simulink subsystem "In_Plane_Model"  (R2025b)
settings: Solver=VariableStepAuto  StartTime=0.0  StopTime=10.0  RelTol=1e-3
undefined symbols (not defined in the file): AeroLiftCff, AeroLongDrgCff, AeroMotoEffctArea, AeroPitchMomentCff, AeroPitchMomentLngth, AeroRltWindAngVect, AeroSideFrcCff, AeroYawMomentCff, aMode, BrkFrntBrkActrBore, BrkFrntBrkActrPrsBpt, BrkFrntBrkPadMeanRadius, BrkFrntBrkTrqTbl, BrkFrntIntrnRadius, BrkFrntKinFricCff, BrkFrntPadNum, BrkFrntShoePinToDrumCntrDst, BrkFrntShoePinToFrcAppDst, BrkFrntShoePinToPadEndAng, BrkFrntShoePinToPadStartAng, BrkFrntStcFricCff, BrkFrntWhlSpdBpt, BrkRearBrkActrBore, BrkRearBrkActrPrsBpt, BrkRearBrkPadMeanRadius, BrkRearBrkTrqTbl, BrkRearIntrnRadius, BrkRearKinFricCff, BrkRearPadNum, BrkRearShoePinToDrumCntrDst, BrkRearShoePinToFrcAppDst, BrkRearShoePinToPadEndAng, BrkRearShoePinToPadStartAng, BrkRearStcFricCff, BrkRearWhlSpdBpt, EnvAbsPrs, EnvAirTemp, FrkFrL0, FrmAng0, g, GasCnst, InitFrkLngth, InitMainFrmPitchAng, InitRearArmPitchAng, InitRearCntctPtchLatVel, InitRearCntctPtchLongVel, InitRearCntctPtchY, InitRearCntctPtchZ, InitRollAng, InitYawAng, MotoFrmLngth, MotoFrmMass, MotoGrvty, MotoLatOfst, MotoLongOfst, MotoLowrFrntFrkMass, MotoPtchOfst, MotoRearArmLngth, MotoRearArmMass, MotoRollOfst ... (+25)
libraries: sm_lib x309, nesl_utility_internal x158, nesl_utility x7, autolibsharedcoupling x6, vehdynlibtire x6, sharedtransform x4, shared6dof x1, matrix_library x1, vehdynlibeomcommon x1
(part 1 of 10)
settings Model: Creator=The MathWorks, Inc.  LastModifiedBy=Omen
settings RTWCC: GPUComputeCapability=3.5

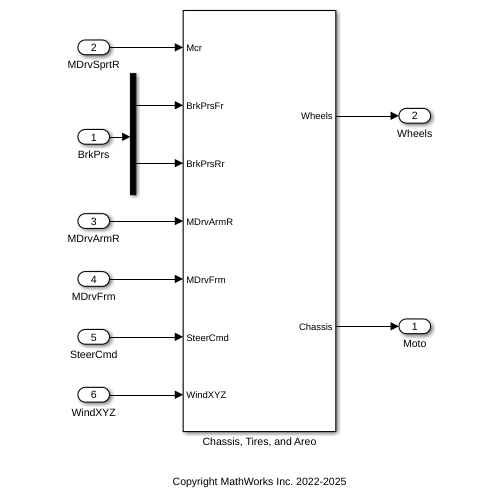
[thumbnail: Simulink's stored preview of the top-level diagram]
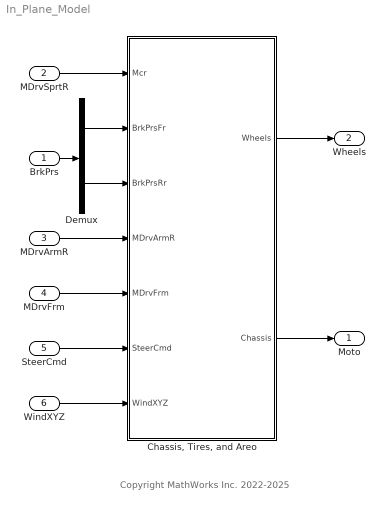
== system In_Plane_Model ==
  note: Copyright MathWorks Inc. 2022-2025
  BrkPrs : Inport
  MDrvSprtR : Inport  Port=2
  MDrvArmR : Inport  Port=3
  MDrvFrm : Inport  Port=4
  SteerCmd : Inport  Port=5
  WindXYZ : Inport  Port=6
  "Chassis, Tires, and Areo" : Subsystem
  Demux : Demux  Outputs=2
  Moto : Outport
  Wheels : Outport  Port=2
  wires:
  BrkPrs/1 -> Demux/1
  "Chassis, Tires, and Areo"/1(Wheels) -> Wheels/1
  Demux/2 -> "Chassis, Tires, and Areo"/3(BrkPrsRr)
  Demux/1 -> "Chassis, Tires, and Areo"/2(BrkPrsFr)
  "Chassis, Tires, and Areo"/2(Chassis) -> Moto/1
  MDrvSprtR/1 -> "Chassis, Tires, and Areo"/1(Mcr)
  MDrvFrm/1 -> "Chassis, Tires, and Areo"/5(MDrvFrm)
  MDrvArmR/1 -> "Chassis, Tires, and Areo"/4(MDrvArmR)
  SteerCmd/1 -> "Chassis, Tires, and Areo"/6(SteerCmd)
  WindXYZ/1 -> "Chassis, Tires, and Areo"/7(WindXYZ)

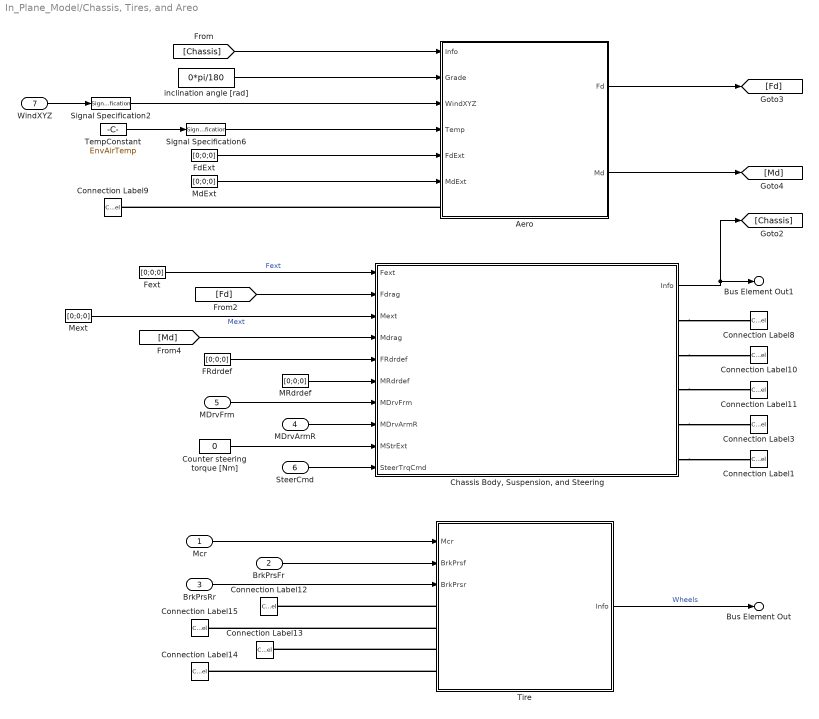
== system In_Plane_Model/Chassis, Tires, and Areo ==
  Mcr : Inport
  BrkPrsFr : Inport  Port=2
  BrkPrsRr : Inport  Port=3
  MDrvArmR : Inport  Port=4
  MDrvFrm : Inport  Port=5
  SteerCmd : Inport  Port=6
  WindXYZ : Inport  Port=7
  Aero : Subsystem  Variant=on  VariantControlMode=label  VariantControl=Choice  LabelModeActiveChoice=None
  "Chassis Body, Suspension, and Steering" : Subsystem
  Connection Label1 : ConnectionLabel  Label=WhlHubFr_B
  Connection Label10 : ConnectionLabel  Label=WhlHubRr_F
  Connection Label11 : ConnectionLabel  Label=WhlHubFr_F
  Connection Label12 : ConnectionLabel  Label=WhlHubFr_B
  Connection Label13 : ConnectionLabel  Label=WhlHubRr_B
  Connection Label14 : ConnectionLabel  Label=WhlHubRr_F
  Connection Label15 : ConnectionLabel  Label=WhlHubFr_F
  Connection Label3 : ConnectionLabel  Label=WhlHubRr_B
  Connection Label8 : ConnectionLabel  Label=AeroFrame_Frm
  Connection Label9 : ConnectionLabel  Label=AeroFrame_Frm
  Counter steering torque [Nm] : Constant  Value=0
  FRdrdef : Constant  Value=[0;0;0]
  FdExt : Constant  Value=[0;0;0]
  Fext : Constant  Value=[0;0;0]
  MRdrdef : Constant  Value=[0;0;0]
  MdExt : Constant  Value=[0;0;0]
  Mext : Constant  Value=[0;0;0]
  Signal Specification2 : SignalSpecification  Unit=m/s
  Signal Specification6 : SignalSpecification  Unit=K
  TempConstant : Constant  Value=EnvAirTemp
  Tire : Subsystem
  inclination angle [rad] : Constant  Value=0*pi/180
  Bus Element Out : Outport  PortName=Wheels
  Bus Element Out1 : Outport  Port=2  PortName=Chassis
  wires:
  SteerCmd/1 -> "Chassis Body, Suspension, and Steering"/10(SteerTrqCmd)
  Counter steering torque [Nm]/1 -> "Chassis Body, Suspension, and Steering"/9(MStrExt)
  MDrvArmR/1 -> "Chassis Body, Suspension, and Steering"/8(MDrvArmR)
  MDrvFrm/1 -> "Chassis Body, Suspension, and Steering"/7(MDrvFrm)
  [Chassis] -> Aero/1(Info)
  "Chassis Body, Suspension, and Steering"/1(Info) -> [Chassis], Bus Element Out1/1
  Tire/1(Info) -> Bus Element Out/1  "Wheels"
  BrkPrsRr/1 -> Tire/3(BrkPrsr)
  Mcr/1 -> Tire/1(Mcr)
  BrkPrsFr/1 -> Tire/2(BrkPrsf)
  MRdrdef/1 -> "Chassis Body, Suspension, and Steering"/6(MRdrdef)
  FRdrdef/1 -> "Chassis Body, Suspension, and Steering"/5(FRdrdef)
  [Md] -> "Chassis Body, Suspension, and Steering"/4(Mdrag)
  [Fd] -> "Chassis Body, Suspension, and Steering"/2(Fdrag)
  Fext/1 -> "Chassis Body, Suspension, and Steering"/1(Fext)  "Fext"
  Mext/1 -> "Chassis Body, Suspension, and Steering"/3(Mext)  "Mext"
  Aero/2(Md) -> [Md]
  Aero/1(Fd) -> [Fd]
  Signal Specification6/1 -> Aero/4(Temp)
  Signal Specification2/1 -> Aero/3(WindXYZ)
  FdExt/1 -> Aero/5(FdExt)
  WindXYZ/1 -> Signal Specification2/1
  inclination angle [rad]/1 -> Aero/2(Grade)
  TempConstant/1 -> Signal Specification6/1
  MdExt/1 -> Aero/6(MdExt)
  connections:
  Tire/LConn3 -- Connection Label13/LConn1
  "Chassis Body, Suspension, and Steering"/RConn4 -- Connection Label3/LConn1
  "Chassis Body, Suspension, and Steering"/RConn2 -- Connection Label10/LConn1
  "Chassis Body, Suspension, and Steering"/RConn3 -- Connection Label11/LConn1
  "Chassis Body, Suspension, and Steering"/RConn1 -- Connection Label8/LConn1
  "Chassis Body, Suspension, and Steering"/RConn5 -- Connection Label1/LConn1
  Tire/LConn4 -- Connection Label14/LConn1
  Tire/LConn1 -- Connection Label12/LConn1
  Tire/LConn2 -- Connection Label15/LConn1
  Aero/LConn1 -- Connection Label9/LConn1

== system In_Plane_Model/Chassis, Tires, and Areo/Aero ==
  Info : Inport
  Grade : Inport  Port=2
  WindXYZ : Inport  Port=3
  Temp : Inport  Port=4
  FdExt : Inport  Port=5
  MdExt : Inport  Port=6
  External : Subsystem  VariantControl=External
  None : Subsystem  VariantControl=None
  Standard Ambient : Subsystem  VariantControl=Standard Ambient
  AeroFrame_Frm : PMIOPort  Side=Left
  Fd : Outport
  Md : Outport  Port=2

== system In_Plane_Model/Chassis, Tires, and Areo/Chassis Body, Suspension, and Steering ==
  Fext : Inport
  Fdrag : Inport  Port=2
  Mext : Inport  Port=3
  Mdrag : Inport  Port=4
  FRdrdef : Inport  Port=5
  MRdrdef : Inport  Port=6
  MDrvFrm : Inport  Port=7
  MDrvArmR : Inport  Port=8
  MStrExt : Inport  Port=9
  SteerTrqCmd : Inport  Port=10
  CHASSIS : Subsystem
  FSusfin : Ground
  MStrDmpin : Ground
  MSusrin : Ground
  Signal routine : Subsystem
  WhlHubFr_F : PMIOPort  Side=Right
  WhlHubRr_F : PMIOPort  Port=2  Side=Right
  AeroFrame_Frm : PMIOPort  Port=3  Side=Right
  WhlHubRr_B : PMIOPort  Port=4  Side=Right
  WhlHubFr_B : PMIOPort  Port=5  Side=Right
  Info : Outport
  wires:
  Mdrag/1 -> [Md], CHASSIS/6(Mdrag)
  Fdrag/1 -> [Fd], CHASSIS/5(Fdrag)  "Fdrag"
  MStrExt/1 -> CHASSIS/8(MStrExt)
  CHASSIS/16(GeomInfo) -> Signal routine/19(GeomInfo)
  MStrDmpin/1 -> CHASSIS/13(MStrDmpin)
  MRdrdef/1 -> CHASSIS/12(MRdrdef)
  FRdrdef/1 -> CHASSIS/11(FRdrdef)
  CHASSIS/15(Q,A,V,P_Rdr) -> Signal routine/18(Q,A,V,P_Rdr)
  FSusfin/1 -> CHASSIS/10(FSusfin)
  MSusrin/1 -> CHASSIS/9(MSusrin)
  CHASSIS/14(Grvty) -> Signal routine/17(Grvty)
  CHASSIS/13(Fext_BF) -> Signal routine/16(Fext_BF)
  CHASSIS/4(WhlFrCpY) -> Signal routine/7(WhlFrCpY)
  Mext/1 -> CHASSIS/2(Mext), [Mext]  "Mext"
  CHASSIS/12(A,V,P_str) -> Signal routine/15(SteerAng)
  CHASSIS/3(WhlRrCpY) -> Signal routine/6(WhlRrCpY)
  SteerTrqCmd/1 -> CHASSIS/7(MSteer)
  [Fd] -> Signal routine/2(Fd)
  [Md] -> Signal routine/3(Md)
  MDrvArmR/1 -> CHASSIS/3(MDrvArmR)  "MDrvArmR"
  MDrvFrm/1 -> CHASSIS/4(MDrvFrm)  "MDrvFrm"
  Signal routine/1(Info) -> Info/1  "ChassisInfo"
  CHASSIS/11(FrkFz) -> Signal routine/14(Frk)
  CHASSIS/10(ShkMy) -> Signal routine/13(Shk)
  CHASSIS/9(Lfrk) -> Signal routine/12(Lfrk)
  CHASSIS/8(A,V,P_FrmAng) -> Signal routine/11(FrmAng)
  CHASSIS/7(ArmRrAng) -> Signal routine/10(ArmRrAng)
  CHASSIS/6(WhlFrCpZ) -> Signal routine/9(WhlFrCpZ)
  CHASSIS/5(WhlRrCpZ) -> Signal routine/8(WhlRrCpZ)
  CHASSIS/2(WhlFrCpX) -> Signal routine/5(WhlFrCpX)
  CHASSIS/1(WhlRrCpX) -> Signal routine/4(WhlRrCpX)
  [Mext] -> Signal routine/1(Mext)
  Fext/1 -> CHASSIS/1(Fext)  "Fext"
  connections:
  CHASSIS/RConn9 -- AeroFrame_Frm/RConn1
  Signal routine/LConn1 -- CHASSIS/RConn1
  Signal routine/LConn2 -- CHASSIS/RConn2
  Signal routine/LConn7 -- CHASSIS/RConn7
  CHASSIS/RConn6 -- Signal routine/LConn6
  CHASSIS/RConn5 -- Signal routine/LConn5
  CHASSIS/RConn3 -- Signal routine/LConn3
  WhlHubRr_F/RConn1 -- CHASSIS/RConn11
  WhlHubFr_F/RConn1 -- CHASSIS/RConn10
  Signal routine/LConn8 -- CHASSIS/RConn8
  WhlHubRr_B/RConn1 -- CHASSIS/LConn1
  Signal routine/LConn4 -- CHASSIS/RConn4
  CHASSIS/LConn2 -- WhlHubFr_B/RConn1

== system In_Plane_Model/Chassis, Tires, and Areo/Tire ==
  Mcr : Inport
  BrkPrsf : Inport  Port=2
  BrkPrsr : Inport  Port=3
  Bus Creator : BusCreator  Inputs=2
  Front Tire : Subsystem  Variant=on  VariantControlMode=label  LabelModeActiveChoice=Linear Front SSC Tire
  MWhf : Ground
  MWhr : Ground
  Mcrf : Ground
  Rear Tire : Subsystem  Variant=on  VariantControlMode=label  LabelModeActiveChoice=Linear Rear SSC Tire
  Terminator{,1..11} (12 alike) : Terminator
  HubJointFr_B : PMIOPort  Side=Left
  HubJointFr_F : PMIOPort  Port=2  Side=Left
  HubJointRr_B : PMIOPort  Port=3  Side=Left
  HubJointRr_F : PMIOPort  Port=4  Side=Left
  Info : Outport
  wires:
  Bus Creator/1 -> Info/1
  Front Tire/4(Fz) -> Terminator2/1  "Fz"
  Mcrf/1 -> Front Tire/2(Mcr)
  Front Tire/2(Fx) -> Terminator/1  "Fx"
  Front Tire/6(My) -> Terminator4/1  "My"
  Front Tire/7(Mz) -> Terminator5/1  "Mz"
  Front Tire/5(Mx) -> Terminator3/1  "Mx"
  Front Tire/1(Info) -> Bus Creator/1  "FrontTire"
  BrkPrsf/1 -> Front Tire/3(BrkPrs)
  Front Tire/3(Fy) -> Terminator1/1  "Fy"
  Rear Tire/3(Fy) -> Terminator7/1  "Fy"
  Rear Tire/2(Fx) -> Terminator6/1  "Fx"
  Rear Tire/4(Fz) -> Terminator8/1  "Fz"
  Rear Tire/7(Mz) -> Terminator11/1  "Mz"
  Rear Tire/5(Mx) -> Terminator9/1  "Mx"
  Rear Tire/6(My) -> Terminator10/1  "My"
  Rear Tire/1(Info) -> Bus Creator/2  "RearTire"
  MWhf/1 -> Front Tire/1(MWh)
  BrkPrsr/1 -> Rear Tire/3(BrkPrs)
  MWhr/1 -> Rear Tire/1(MWh)
  Mcr/1 -> Rear Tire/2(Mcr)
  connections:
  Front Tire/LConn1 -- HubJointFr_B/RConn1
  Front Tire/LConn2 -- HubJointFr_F/RConn1
  Rear Tire/LConn2 -- HubJointRr_F/RConn1
  Rear Tire/LConn1 -- HubJointRr_B/RConn1

== system In_Plane_Model/Chassis, Tires, and Areo/Aero/External ==
  FdExt : Inport
  MdExt : Inport  Port=2
  Fd : Outport
  Md : Outport  Port=2
  wires:
  MdExt/1 -> Md/1
  FdExt/1 -> Fd/1

== system In_Plane_Model/Chassis, Tires, and Areo/Aero/None ==
  Constant : Constant  Value=[0 0 0]
  Constant1 : Constant  Value=[0 0 0]
  Fd : Outport
  Md : Outport  Port=2
  wires:
  Constant/1 -> Fd/1
  Constant1/1 -> Md/1

== system In_Plane_Model/Chassis, Tires, and Areo/Aero/Standard Ambient ==
  Info : Inport
  Grade : Inport  Port=2  Unit=rad
  WindXYZ : Inport  Port=3  PortDimensions=3
  Temp : Inport  Port=4
  Bus Selector6 : BusSelector  OutputSignals=Frame.InertFrm.Cg.Ang.theta
  Drag Force : Subsystem  mask{A=AeroMotoEffctArea, beta_w=AeroRltWindAngVect, Cd=AeroLongDrgCff, Cs=AeroSideFrcCff, Cl=AeroLiftCff, Cpm=AeroPitchMomentCff, Lcpm=AeroPitchMomentLngth, Crm=[0,0], Cym=AeroYawMomentCff, R=GasCnst, Pabs=EnvAbsPrs}
      mask prompts: A "Effective area, A [m^s2]:"; beta_w "Relative wind angle vector, beta_w [rad]:"; Cd "Longitudinal drag coefficient, Cd [-]:"; Cs "Side force coefficient data, Cs [-]:"; Cl "Lift coefficient, Cl [-]:"; Cpm "Pitch moment coefficient, Cpm [-]:"; Lcpm "Pitch moment length, Lcpm"; Crm "Roll moment coefficient data, Crm [-]:"; Cym "Yaw moment coefficient data, Cym [-]:"; R "Gas constant, R [J/(kg*K)]:"; Pabs "Absoulte pressure, Pabs [Pa]:"
  Mux6 : Mux  Inputs=3
  Sensor_Frm : Subsystem
  Subtract : Sum  Inputs=--
  Unary Minus : UnaryMinus
  Unary Minus1 : UnaryMinus
  rotation : Subsystem  TreatAsAtomicUnit=on  mask(Rotation){aMode=aMode}
  AeroFrame_Frm : PMIOPort  Side=Left
  Fd : Outport
  Md : Outport  Port=2
  wires:
  Sensor_Frm/3(Vz_vf) -> Mux6/3
  Temp/1 -> Drag Force/3(T)
  Sensor_Frm/1(Vx_vf) -> Mux6/1
  Mux6/1 -> Drag Force/1(Body Axis Vel)
  WindXYZ/1 -> rotation/1(X)
  Bus Selector6/1 -> Subtract/1  "<theta>"
  Sensor_Frm/2(Vy_vf) -> Mux6/2
  Info/1 -> Bus Selector6/1
  Drag Force/1(Fd) -> Unary Minus1/1
  Drag Force/2(Md) -> Unary Minus/1
  Subtract/1 -> rotation/2(theta)
  Grade/1 -> Subtract/2
  rotation/1(x) -> Drag Force/2(Body Axis Wind)
  Unary Minus1/1 -> Fd/1
  Unary Minus/1 -> Md/1
  connections:
  AeroFrame_Frm/RConn1 -- Sensor_Frm/LConn1

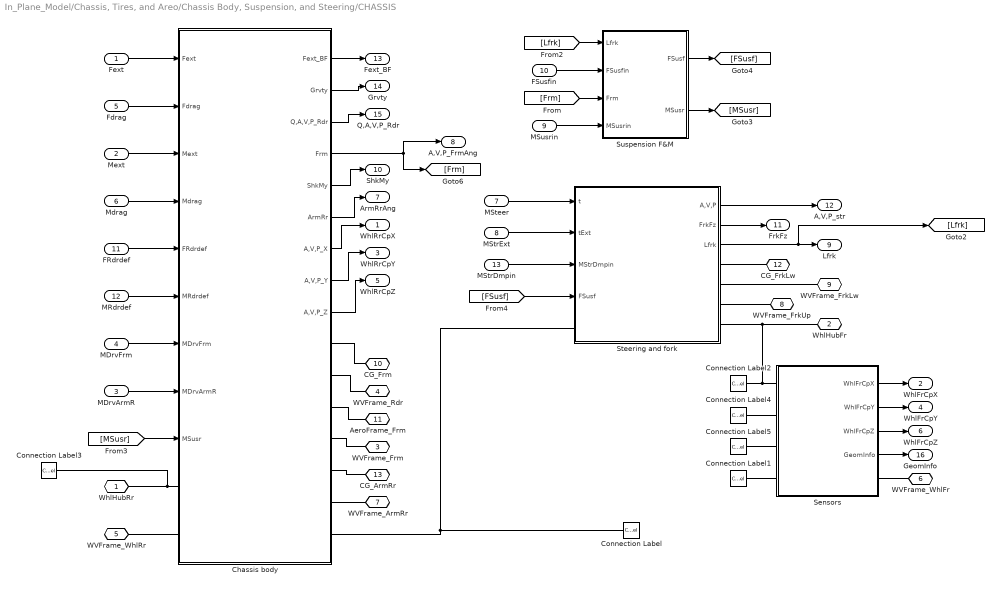
== system In_Plane_Model/Chassis, Tires, and Areo/Chassis Body, Suspension, and Steering/CHASSIS ==
  Fext : Inport
  Mext : Inport  Port=2
  MDrvArmR : Inport  Port=3
  MDrvFrm : Inport  Port=4
  Fdrag : Inport  Port=5
  Mdrag : Inport  Port=6
  MSteer : Inport  Port=7
  MStrExt : Inport  Port=8
  MSusrin : Inport  Port=9
  FSusfin : Inport  Port=10
  FRdrdef : Inport  Port=11
  MRdrdef : Inport  Port=12
  MStrDmpin : Inport  Port=13
  Chassis body : Subsystem
  Connection Label : ConnectionLabel  Label=pivo
  Connection Label1 : ConnectionLabel  Label=pivo
  Connection Label2 : ConnectionLabel  Label=HubFr
  Connection Label3 : ConnectionLabel  Label=HubRr
  Connection Label4 : ConnectionLabel  Label=HubRr
  Connection Label5 : ConnectionLabel  Label=HubFr
  Sensors : Subsystem
  Steering and fork : Subsystem
  Suspension F&M : Subsystem
  WhlHubRr : PMIOPort  Side=Left
  WhlHubFr : PMIOPort  Port=2  Side=Left
  WVFrame_Frm : PMIOPort  Port=3  Side=Right
  WVFrame_Rdr : PMIOPort  Port=4  Side=Right
  WVFrame_WhlRr : PMIOPort  Port=5  Side=Right
  WVFrame_WhlFr : PMIOPort  Port=6  Side=Right
  WVFrame_ArmRr : PMIOPort  Port=7  Side=Right
  WVFrame_FrkUp : PMIOPort  Port=8  Side=Right
  WVFrame_FrkLw : PMIOPort  Port=9  Side=Right
  CG_Frm : PMIOPort  Port=10  Side=Right
  AeroFrame_Frm : PMIOPort  Port=11  Side=Right
  CG_FrkLw : PMIOPort  Port=12  Side=Right
  CG_ArmRr : PMIOPort  Port=13  Side=Right
  WhlRrCpX : Outport
  WhlFrCpX : Outport  Port=2
  WhlRrCpY : Outport  Port=3
  WhlFrCpY : Outport  Port=4
  WhlRrCpZ : Outport  Port=5
  WhlFrCpZ : Outport  Port=6
  ArmRrAng : Outport  Port=7
  A,V,P_FrmAng : Outport  Port=8
  Lfrk : Outport  Port=9
  ShkMy : Outport  Port=10
  FrkFz : Outport  Port=11
  A,V,P_str : Outport  Port=12
  Fext_BF : Outport  Port=13
  Grvty : Outport  Port=14
  Q,A,V,P_Rdr : Outport  Port=15
  GeomInfo : Outport  Port=16
  wires:
  Chassis body/9(A,V,P_Z) -> WhlRrCpZ/1
  Chassis body/8(A,V,P_Y) -> WhlRrCpY/1
  Chassis body/7(A,V,P_X) -> WhlRrCpX/1
  Chassis body/6(ArmRr) -> ArmRrAng/1
  Chassis body/5(ShkMy) -> ShkMy/1
  Chassis body/3(Q,A,V,P_Rdr) -> Q,A,V,P_Rdr/1
  Chassis body/2(Grvty) -> Grvty/1
  Chassis body/1(Fext_BF) -> Fext_BF/1
  [MSusr] -> Chassis body/9(MSusr)
  MDrvArmR/1 -> Chassis body/8(MDrvArmR)
  MDrvFrm/1 -> Chassis body/7(MDrvFrm)
  MRdrdef/1 -> Chassis body/6(MRdrdef)
  FRdrdef/1 -> Chassis body/5(FRdrdef)
  Mdrag/1 -> Chassis body/4(Mdrag)
  Mext/1 -> Chassis body/3(Mext)
  Fdrag/1 -> Chassis body/2(Fdrag)
  Fext/1 -> Chassis body/1(Fext)
  Chassis body/4(Frm) -> A,V,P_FrmAng/1, [Frm]
  Steering and fork/2(FrkFz) -> FrkFz/1
  Steering and fork/1(A,V,P) -> A,V,P_str/1
  [FSusf] -> Steering and fork/4(FSusf)
  MStrDmpin/1 -> Steering and fork/3(MStrDmpin)
  MStrExt/1 -> Steering and fork/2(tExt)
  MSteer/1 -> Steering and fork/1(t)
  Steering and fork/3(Lfrk) -> Lfrk/1, [Lfrk]
  Sensors/4(GeomInfo) -> GeomInfo/1
  Sensors/3(WhlFrCpZ) -> WhlFrCpZ/1
  Sensors/2(WhlFrCpY) -> WhlFrCpY/1
  Sensors/1(WhlFrCpX) -> WhlFrCpX/1
  Suspension F&M/2(MSusr) -> [MSusr]
  Suspension F&M/1(FSusf) -> [FSusf]
  MSusrin/1 -> Suspension F&M/4(MSusrin)
  [Frm] -> Suspension F&M/3(Frm)
  FSusfin/1 -> Suspension F&M/2(FSusfin)
  [Lfrk] -> Suspension F&M/1(Lfrk)
  connections:
  WVFrame_WhlRr/RConn1 -- Chassis body/LConn2
  Chassis body/RConn6 -- WVFrame_ArmRr/RConn1
  Chassis body/RConn5 -- CG_ArmRr/RConn1
  WVFrame_Frm/RConn1 -- Chassis body/RConn4
  AeroFrame_Frm/RConn1 -- Chassis body/RConn3
  Chassis body/RConn2 -- WVFrame_Rdr/RConn1
  CG_Frm/RConn1 -- Chassis body/RConn1
  Chassis body/LConn1 -- WhlHubRr/RConn1 -- Connection Label3/LConn1
  Chassis body/RConn7 -- Steering and fork/LConn1 -- Connection Label/LConn1
  Steering and fork/RConn3 -- WVFrame_FrkUp/RConn1
  Steering and fork/RConn2 -- WVFrame_FrkLw/RConn1
  Steering and fork/RConn1 -- CG_FrkLw/RConn1
  Sensors/LConn4 -- Connection Label1/LConn1
  Sensors/LConn3 -- Connection Label5/LConn1
  Connection Label4/LConn1 -- Sensors/LConn2
  Sensors/RConn1 -- WVFrame_WhlFr/RConn1
  WhlHubFr/RConn1 -- Steering and fork/RConn4 -- Sensors/LConn1 -- Connection Label2/LConn1

== system In_Plane_Model/Chassis, Tires, and Areo/Chassis Body, Suspension, and Steering/Signal routine ==
  Mext : Inport
  Fd : Inport  Port=2
  Md : Inport  Port=3
  WhlRrCpX : Inport  Port=4
  WhlFrCpX : Inport  Port=5
  WhlRrCpY : Inport  Port=6
  WhlFrCpY : Inport  Port=7
  WhlRrCpZ : Inport  Port=8
  WhlFrCpZ : Inport  Port=9
  ArmRrAng : Inport  Port=10
  FrmAng : Inport  Port=11
  Lfrk : Inport  Port=12
  Shk : Inport  Port=13
  Frk : Inport  Port=14
  SteerAng : Inport  Port=15
  Fext_BF : Inport  Port=16
  Grvty : Inport  Port=17
  Q,A,V,P_Rdr : Inport  Port=18
  GeomInfo : Inport  Port=19
  Ancillary_sub : Subsystem
  Bus Creator12 : BusCreator  Inputs=8
  Geom : Subsystem
  Info_sub : Subsystem
      settings: PortSchema="{\"entries\":[{\"content\":{\"sides\":[{\"content\":{\"connectorIds\":[\"LConn1\",\"In1\",\"In2\",\"In3\",\"In4\",\"In5\",\"In6\"]},\"type\":\"ConnectorPlacement.EquallySpacedRectSide\",\"uuid\":\"4ecbd4ae-1654-4997-9989-88e0c36cbdd4\"},{\"content\":{\"connectorIds\":[\"Out1\"],\"side\":\"RIGHT\"},\"type\":\"ConnectorPlacement.EquallySpacedRectSide\",\"uuid\":\"f0d457c7-b83f-4f98-93cd-bb44a09287fe\"},{\"content\":{\"side\":\"TOP\"},\"type\":\"ConnectorPlacement.EquallySpacedRectSide\",\"uuid\":\"b5011b05-5a79-4eec-86a1-ae828fee4e52\"}]},\"type\":\"ConnectorPlacement.EquallySpacedConnector\",\"uuid\":\"9f66f65c-095d-49d5-95d1-46193111b387\"}],\"packageUris\":[\"http://schema.mathworks.com/mf0/Connector/R2020b\"],\"version\":\"1.0\"}"
  Subsystem Info Busses : Subsystem
  WVFrame_Frm : PMIOPort  Side=Left
  WVFrame_Rdr : PMIOPort  Port=2  Side=Left
  WVFrame_WhlRr : PMIOPort  Port=3  Side=Left
  WVFrame_WhlFr : PMIOPort  Port=4  Side=Left
  WVFrame_ArmRr : PMIOPort  Port=5  Side=Left
  WVFrame_FrkUp : PMIOPort  Port=6  Side=Left
  WVFrame_FrkLw : PMIOPort  Port=7  Side=Left
  CG_Frm : PMIOPort  Port=8  Side=Left
  Info : Outport
  wires:
  Subsystem Info Busses/7(Rdr) -> Bus Creator12/7  "Rdr"
  Geom/1(Geom) -> Bus Creator12/8  "Geom"
  GeomInfo/1 -> Geom/1(GeomInfo)
  Q,A,V,P_Rdr/1 -> Ancillary_sub/13(Q,A,V,P_Rdr)
  Fext_BF/1 -> Info_sub/1(Fext_BF)
  FrmAng/1 -> Ancillary_sub/8(FrmAng)
  Subsystem Info Busses/6(Steer) -> Bus Creator12/6  "Steer"
  SteerAng/1 -> Ancillary_sub/12(SteerAng), Geom/2(SteerAng)
  WhlFrCpY/1 -> Ancillary_sub/4(WhlFrCpY)
  WhlRrCpY/1 -> Ancillary_sub/3(WhlRrCpY)
  Subsystem Info Busses/4(Fork) -> Bus Creator12/4  "Fork"
  Info_sub/1(Frame) -> Bus Creator12/1  "Frame"
  Subsystem Info Busses/1(Frm) -> Info_sub/6(Genrl)  "Genrl"
  Subsystem Info Busses/5(Susp) -> Bus Creator12/5  "Susp"
  Subsystem Info Busses/3(RearArm) -> Bus Creator12/3  "RearArm"
  Subsystem Info Busses/2(Whl) -> Bus Creator12/2  "Whl"
  Fd/1 -> Info_sub/3(Fd)
  Md/1 -> Info_sub/4(Md)
  Frk/1 -> Ancillary_sub/11(Frk)
  Lfrk/1 -> Ancillary_sub/9(Lfrk)
  Shk/1 -> Ancillary_sub/10(Shk)
  WhlFrCpZ/1 -> Ancillary_sub/6(WhlFrCpZ)
  ArmRrAng/1 -> Ancillary_sub/7(ArmRrAng)
  WhlRrCpZ/1 -> Ancillary_sub/5(WhlRrCpZ)
  WhlFrCpX/1 -> Ancillary_sub/2(WhlFrCpX)
  WhlRrCpX/1 -> Ancillary_sub/1(WhlRrCpX)
  Bus Creator12/1 -> Info/1  "Info"
  Grvty/1 -> Info_sub/2(Fg)
  Mext/1 -> Info_sub/5(Mext)
  Ancillary_sub/1(Ancillary) -> Subsystem Info Busses/1(Info In)  "Ancillary"
  connections:
  Ancillary_sub/LConn7 -- WVFrame_Frm/RConn1
  WVFrame_Rdr/RConn1 -- Ancillary_sub/LConn4
  Ancillary_sub/LConn6 -- WVFrame_FrkLw/RConn1
  WVFrame_WhlRr/RConn1 -- Ancillary_sub/LConn1
  Ancillary_sub/LConn2 -- WVFrame_WhlFr/RConn1
  Ancillary_sub/LConn3 -- WVFrame_ArmRr/RConn1
  Ancillary_sub/LConn5 -- WVFrame_FrkUp/RConn1
  CG_Frm/RConn1 -- Info_sub/LConn1

== system In_Plane_Model/Chassis, Tires, and Areo/Tire/Front Tire ==
  note: 1) Add Subsystem or Model blocks as valid variant choices.
      | 2) You cannot connect blocks at this level. At simulation, connectivity is automatically
      | determined, based on the active variant and port name matching.
  MWh : Inport
  Mcr : Inport  Port=2
  BrkPrs : Inport  Port=3
  Linear Front SSC Tire : Subsystem  VariantControl=Linear Front SSC Tire  mask{BrakeTypePanel=Disc, FrictionTypePanel=Linear, VDeflectionTypePanel=Simple spring and damper, kx=TireFrntBrkDrvStf, kyl=TireFrntCrnrStf, kyc=TireFrntCamberStf, mu_static=BrkFrntStcFricCff, mu_kinetic=BrkFrntKinFricCff, drum_abore=BrkFrntBrkActrBore, drum_a=BrkFrntShoePinToDrumCntrDst, drum_c=BrkFrntShoePinToFrcAppDst, drum_r=BrkFrntIntrnRadius, drum_theta1=BrkFrntShoePinToPadStartAng, drum_theta2=BrkFrntShoePinToPadEndAng, disk_abore=BrkFrntBrkActrBore, Rm=BrkFrntBrkPadMeanRadius, num_pads=BrkFrntPadNum, brake_p_bpt=BrkFrntBrkActrPrsBpt, brake_n_bpt=BrkFrntWhlSpdBpt, f_brake_t=BrkFrntBrkTrqTbl, kz=TireFrntVertStf, cz=TireFrntVertDamp, WhlMass=TireFrntWhlMass, whlInert=TireFrntWhlInert, RWhl=TireFrntWhlRadius, omegao=-InitRearCntctPtchLongVel/TireFrntWhlRadius, aMode=2}
      mask prompts: BrakeTypePanel "Brake type:"; FrictionTypePanel "Friction model type:"; VDeflectionTypePanel "Vertical Deflection model type:"; kx "Braking/Driving stiffness, kx [-]:"; kyl "Cornering stiffness, kyl [-]:"; kyc "Camber stiffness, kyc [-]:"; mu_static "Static friction coefficient, mu_static []:"; mu_kinetic "Kinetic friction coefficient, mu_kinetic []:"; drum_abore "Drum brake actuator bore, drum_abore [m]:"; drum_a "Shoe pin to drum center distance, drum_a [m]:"; drum_c "Shoe pin center to force application point distance, drum_c [m]:"; drum_r "Drum internal radius, drum_r [m]:"; drum_theta1 "Shoe pin to pad start angle, drum_theta1 [deg]:"; drum_theta2 "Shoe pin to pad end angle, drum_theta2 [deg]:"; disk_abore "Disc brake actuator bore, disk_abore [m]:"; Rm "Brake pad mean radius, Rm [m]:"; num_pads "Number of brake pads, num_pads []:"; brake_p_bpt "Brake actuator pressure breakpoints, brake_p_bpt [bar]:"; brake_n_bpt "Wheel speed breakpoints, brake_n_bpt [rpm]:"; f_brake_t "Brake torque map, f_brake_t [Nm]:"; kz "Vertical stiffness, kz [N/m]:"; cz "Vertical damping, cz [Ns/m]:"; WhlMass "Mass, WhlMass [kg]:"; whlInert "Wheel Inertia tensor, whlInert [Kg*m^2]:"; RWhl "Unloaded radius, RWhl [m]:"; omegao "Wheel initial angular velocity, omegao [rad/s]:"
      settings: LibrarySourceBlock=|
      | MotoLongBTReferenceApplication/Motorcycle Vehicle/Body, Suspension, Wheels/Simscape Multibody Lateral/Simscape Multibody model/Wheels1/Linear Front tire
      | (Simscape Multibody)
      mask TypeOptions BrakeTypePanel: None | Disc | Drum | Mapped | External
      mask Callback BrakeTypePanel:
      | maskObj = Simulink.Mask.get(gcb);
      | 
      | Type_tmp = maskObj.getParameter('BrakeTypePanel');
      | Type     = Type_tmp.Value;
      | 
      | GeneralGroup = maskObj.getDialogControl('BrakeGeneralGroup');
      | DrumGroup    = maskObj.getDialogControl('BrakeDrumGroup');
      | DiscGroup    = maskObj.getDialogControl('BrakeDiscGroup');
      | MappedGroup  = maskObj.getDialogControl('BrakeMappedGroup');
      | 
      | BrakePanel = maskObj.getDialogControl('BrakeGroup');
      | 
      | switch Type
      |     case 'External'
      |     set_param([gcb,'/Brake model'],'LabelModeActiveChoice', 'External');
      |     BrakePanel.Visible   = 'off';
      |     InputConnector('MBrkin','on','Ground','');
      |     InputConnector('BrkPrs','off','Ground','');
      |     case 'Disc'
      |     set_param([gcb,'/Brake model'],'LabelModeActiveChoice', 'MW Brake');
      |     set_param([gcb,'/Brake model/MW Brake/Brakes'],'LabelModeActiveChoice', 'Disk');
      |     BrakePanel.Visible   = 'on';
      |     GeneralGroup.Visible = 'on';
      |     DrumGroup.Visible    = 'off';
      |     DiscGroup.Visible    = 'on';
      |     MappedGroup.Visible  = 'off';
      |     InputConnector('MBrkin','off','Ground','');
      |     InputConnector('BrkPrs','on','Ground','');
      |     case 'Drum'
      |     set_param([gcb,'/Brake model'],'LabelModeActiveChoice', 'MW Brake');
      |     set_param([gcb,'/Brake model/MW Brake/Brakes'],'LabelModeActiveChoice', Type);
      |     BrakePanel.Visible   = 'on';
      |     GeneralGroup.Visible = 'on';
      |     DrumGroup.Visible    = 'on';
      |     DiscGroup.Visible    = 'off';
      |     MappedGroup.Visible  = 'off';
      |     InputConnector('MBrkin','off','Ground','');
      |     InputConnector('BrkPrs','on','Ground','');
      |     case 'Mapped'
      |     set_param([gcb,'/Brake model'],'LabelModeActiveChoice', 'MW Brake');
      |     set_param([gcb,'/Brake model/MW Brake/Brakes'],'LabelModeActiveChoice', Type);
      |     BrakePanel.Visible   = 'on';
      |     GeneralGroup.Visible = 'on';
      |     DrumGroup.Visible    = 'off';
      |     DiscGroup.Visible    = 'off';
      |     MappedGroup.Visible  = 'on';
      |     InputConnector('MBrkin','off','Ground','');
      |     InputConnector('BrkPrs','on','Ground','');
      |     case 'None'
      |     set_param([gcb,'/Brake model'],'LabelModeActiveChoice', 'MW Brake');
      |     set_param([gcb,'/Brake model/MW Brake/Brakes'],'LabelModeActiveChoice', Type);
      |     BrakePanel.Visible = 'off';
      |     InputConnector('MBrkin','off','Ground','');
      |     InputConnector('BrkPrs','off','Ground','');
      | end
      mask TypeOptions FrictionTypePanel: Linear | External
      mask Callback FrictionTypePanel:
      | maskObj = Simulink.Mask.get(gcb);
      | 
      | Type_tmp = maskObj.getParameter('FrictionTypePanel');
      | Type     = Type_tmp.Value;
      | 
      | Group = maskObj.getDialogControl('FrictionModelGroup');
      | 
      | switch Type
      |     case 'Linear'
      |     set_param([gcb,'/Friction model'],'LabelModeActiveChoice', 'Linear');
      |     Group.Visible = 'on';
      |     InputConnector('Fxin','off','Ground','');
      |     InputConnector('Fyin','off','Ground','');
      |     InputConnector('Mxin','off','Ground','');
      |     InputConnector('Myin','off','Ground','');
      |     InputConnector('Mzin','off','Ground','');
      |     case 'External'
      |     set_param([gcb,'/Friction model'],'LabelModeActiveChoice', 'External');
      |     Group.Visible = 'off';
      |     InputConnector('Fxin','on','Ground','');
      |     InputConnector('Fyin','on','Ground','');
      |     InputConnector('Mxin','on','Ground','');
      |     InputConnector('Myin','on','Ground','');
      |     InputConnector('Mzin','on','Ground','');
      | end
      mask TypeOptions VDeflectionTypePanel: Simple spring and damper | External
      mask Callback VDeflectionTypePanel:
      | maskObj = Simulink.Mask.get(gcb);
      | 
      | Type_tmp = maskObj.getParameter('VDeflectionTypePanel');
      | Type     = Type_tmp.Value;
      | 
      | Group = maskObj.getDialogControl('VDeflectionModelGroup');
      | 
      | switch Type
      |     case 'Simple spring and damper'
      |     set_param([gcb,'/Contact model'],'LabelModeActiveChoice', 'Simple spring and damper');
      |     Group.Visible = 'on';
      |     InputConnector('Fzin','off','Ground','');
      |     case 'External'
      |     set_param([gcb,'/Contact model'],'LabelModeActiveChoice', 'External');
      |     Group.Visible = 'off';
      |     InputConnector('Fzin','on','Ground','');
      | end
      mask DialogControl BlockOptionsPanel Prompt: Block Options
      mask DialogControl FrictionModelPanel Prompt: Friction model
      mask DialogControl LinearTireModelGroup Prompt: Linear tire model
      mask DialogControl LinLongPanel Prompt: Longitudinal
      mask DialogControl LinLateralPanel Prompt: Lateral
      mask DialogControl BrakeSubPanel Prompt: Brake
      mask DialogControl BrakeGeneralGroup Prompt: General
      mask DialogControl BrakeDrumGroup Prompt: Drum Brake
      mask DialogControl BrakeDiscGroup Prompt: Disc Brake
      mask DialogControl BrakeMappedGroup Prompt: Mapped Brake
      mask DialogControl PlotBrakeTorqueMapButton Prompt: Plot brake torque map
      mask DialogControl PlotBrakeTorqueMapButton Callback:
      | maskObj = Simulink.Mask.get(gcb);
      | tmp = maskObj.getParameter('brake_p_bpt');
      | brake_p_bpt = str2num(tmp.Value);
      | tmp = maskObj.getParameter('brake_n_bpt');
      | brake_n_bpt = str2num(tmp.Value);
      | tmp = maskObj.getParameter('f_brake_t');
      | f_brake_t = str2num(tmp.Value);
      | 
      | figure;
      | surf(brake_p_bpt, brake_n_bpt, f_brake_t');
      | xlabel('Applied brake pressure [bar]');
      | ylabel('Wheel speed [rpm]');
      | zlabel('Brake torque [N*m]');
      | title('Brake torque vs applied pressure and wheel speed');
      mask DialogControl VDeflectionSubPanel Prompt: Vertical Deflection
      mask DialogControl VerticalModelGroup Prompt: Vertical deflection model
      mask DialogControl MassParameterPanel Prompt: Mass parameters
      mask DialogControl DimensionParameterPanel Prompt: Dimension parameters
      mask DialogControl InitialConditionPanel Prompt: Initial condition
  HubJoint_B : PMIOPort  Side=Left
  HubJoint_F : PMIOPort  Port=2  Side=Left
  Info : Outport
  Fx : Outport  Port=2
  Fy : Outport  Port=3
  Fz : Outport  Port=4
  Mx : Outport  Port=5
  My : Outport  Port=6
  Mz : Outport  Port=7

== system In_Plane_Model/Chassis, Tires, and Areo/Tire/Rear Tire ==
  note: 1) Add Subsystem or Model blocks as valid variant choices.
      | 2) You cannot connect blocks at this level. At simulation, connectivity is automatically
      | determined, based on the active variant and port name matching.
  MWh : Inport
  Mcr : Inport  Port=2
  BrkPrs : Inport  Port=3
  Linear Rear SSC Tire : Subsystem  VariantControl=Linear Rear SSC Tire  mask{BrakeTypePanel=Disc, FrictionTypePanel=Linear, VDeflectionTypePanel=Simple spring and damper, kx=TireRearBrkDrvStf, kyl=TireRearCrnrStf, kyc=TireRearCamberStf, mu_static=BrkRearStcFricCff, mu_kinetic=BrkRearKinFricCff, drum_abore=BrkRearBrkActrBore, drum_a=BrkRearShoePinToDrumCntrDst, drum_c=BrkRearShoePinToFrcAppDst, drum_r=BrkRearIntrnRadius, drum_theta1=BrkRearShoePinToPadStartAng, drum_theta2=BrkRearShoePinToPadEndAng, disk_abore=BrkRearBrkActrBore, Rm=BrkRearBrkPadMeanRadius, num_pads=BrkRearPadNum, brake_p_bpt=BrkRearBrkActrPrsBpt, brake_n_bpt=BrkRearWhlSpdBpt, f_brake_t=BrkRearBrkTrqTbl, kz=TireRearVertStf, cz=TireRearVertDamp, WhlMass=TireRearWhlMass, whlInert=TireRearWhlInert, RWhl=TireRearWhlRadius, omegao=-InitRearCntctPtchLongVel/TireRearWhlRadius, aMode=2}
      mask prompts: BrakeTypePanel "Brake type:"; FrictionTypePanel "Friction model type:"; VDeflectionTypePanel "Vertical Deflection model type:"; kx "Braking/Driving stiffness, kx [-]:"; kyl "Cornering stiffness, kyl [-]:"; kyc "Camber stiffness, kyc [-]:"; mu_static "Static friction coefficient, mu_static []:"; mu_kinetic "Kinetic friction coefficient, mu_kinetic []:"; drum_abore "Drum brake actuator bore, drum_abore [m]:"; drum_a "Shoe pin to drum center distance, drum_a [m]:"; drum_c "Shoe pin center to force application point distance, drum_c [m]:"; drum_r "Drum internal radius, drum_r [m]:"; drum_theta1 "Shoe pin to pad start angle, drum_theta1 [deg]:"; drum_theta2 "Shoe pin to pad end angle, drum_theta2 [deg]:"; disk_abore "Disc brake actuator bore, disk_abore [m]:"; Rm "Brake pad mean radius, Rm [m]:"; num_pads "Number of brake pads, num_pads []:"; brake_p_bpt "Brake actuator pressure breakpoints, brake_p_bpt [bar]:"; brake_n_bpt "Wheel speed breakpoints, brake_n_bpt [rpm]:"; f_brake_t "Brake torque map, f_brake_t [Nm]:"; kz "Vertical stiffness, kz [N/m]:"; cz "Vertical damping, cz [Ns/m]:"; WhlMass "Mass, WhlMass [kg]:"; whlInert "Wheel Inertia tensor, whlInert [Kg*m^2]:"; RWhl "Unloaded radius, RWhl [m]:"; omegao "Wheel initial angular velocity, omegao [rad/s]:"
      settings: LibrarySourceBlock=|
      | MotoLongBTReferenceApplication/Motorcycle Vehicle/Body, Suspension, Wheels/Simscape Multibody Lateral/Simscape Multibody model/Wheels1/Linear Rear tire
      | (Simscape Multibody)
      mask TypeOptions BrakeTypePanel: None | Disc | Drum | Mapped | External
      mask Callback BrakeTypePanel:
      | maskObj = Simulink.Mask.get(gcb);
      | 
      | Type_tmp = maskObj.getParameter('BrakeTypePanel');
      | Type     = Type_tmp.Value;
      | 
      | GeneralGroup = maskObj.getDialogControl('BrakeGeneralGroup');
      | DrumGroup    = maskObj.getDialogControl('BrakeDrumGroup');
      | DiscGroup    = maskObj.getDialogControl('BrakeDiscGroup');
      | MappedGroup  = maskObj.getDialogControl('BrakeMappedGroup');
      | 
      | BrakePanel = maskObj.getDialogControl('BrakeGroup');
      | 
      | switch Type
      |     case 'External'
      |     set_param([gcb,'/Brake model'],'LabelModeActiveChoice', 'External');
      |     BrakePanel.Visible   = 'off';
      |     InputConnector('MBrkin','on','Ground','');
      |     InputConnector('BrkPrs','off','Ground','');
      |     case 'Disc'
      |     set_param([gcb,'/Brake model'],'LabelModeActiveChoice', 'MW Brake');
      |     set_param([gcb,'/Brake model/MW Brake/Brakes'],'LabelModeActiveChoice', 'Disk');
      |     BrakePanel.Visible   = 'on';
      |     GeneralGroup.Visible = 'on';
      |     DrumGroup.Visible    = 'off';
      |     DiscGroup.Visible    = 'on';
      |     MappedGroup.Visible  = 'off';
      |     InputConnector('MBrkin','off','Ground','');
      |     InputConnector('BrkPrs','on','Ground','');
      |     case 'Drum'
      |     set_param([gcb,'/Brake model'],'LabelModeActiveChoice', 'MW Brake');
      |     set_param([gcb,'/Brake model/MW Brake/Brakes'],'LabelModeActiveChoice', Type);
      |     BrakePanel.Visible   = 'on';
      |     GeneralGroup.Visible = 'on';
      |     DrumGroup.Visible    = 'on';
      |     DiscGroup.Visible    = 'off';
      |     MappedGroup.Visible  = 'off';
      |     InputConnector('MBrkin','off','Ground','');
      |     InputConnector('BrkPrs','on','Ground','');
      |     case 'Mapped'
      |     set_param([gcb,'/Brake model'],'LabelModeActiveChoice', 'MW Brake');
      |     set_param([gcb,'/Brake model/MW Brake/Brakes'],'LabelModeActiveChoice', Type);
      |     BrakePanel.Visible   = 'on';
      |     GeneralGroup.Visible = 'on';
      |     DrumGroup.Visible    = 'off';
      |     DiscGroup.Visible    = 'off';
      |     MappedGroup.Visible  = 'on';
      |     InputConnector('MBrkin','off','Ground','');
      |     InputConnector('BrkPrs','on','Ground','');
      |     case 'None'
      |     set_param([gcb,'/Brake model'],'LabelModeActiveChoice', 'MW Brake');
      |     set_param([gcb,'/Brake model/MW Brake/Brakes'],'LabelModeActiveChoice', Type);
      |     BrakePanel.Visible = 'off';
      |     InputConnector('MBrkin','off','Ground','');
      |     InputConnector('BrkPrs','off','Ground','');
      | end
      mask TypeOptions FrictionTypePanel: Linear | External
      mask Callback FrictionTypePanel:
      | maskObj = Simulink.Mask.get(gcb);
      | 
      | Type_tmp = maskObj.getParameter('FrictionTypePanel');
      | Type     = Type_tmp.Value;
      | 
      | Group = maskObj.getDialogControl('FrictionModelGroup');
      | 
      | switch Type
      |     case 'Linear'
      |     set_param([gcb,'/Friction model'],'LabelModeActiveChoice', 'Linear');
      |     Group.Visible = 'on';
      |     InputConnector('Fxin','off','Ground','');
      |     InputConnector('Fyin','off','Ground','');
      |     InputConnector('Mxin','off','Ground','');
      |     InputConnector('Myin','off','Ground','');
      |     InputConnector('Mzin','off','Ground','');
      |     case 'External'
      |     set_param([gcb,'/Friction model'],'LabelModeActiveChoice', 'External');
      |     Group.Visible = 'off';
      |     InputConnector('Fxin','on','Ground','');
      |     InputConnector('Fyin','on','Ground','');
      |     InputConnector('Mxin','on','Ground','');
      |     InputConnector('Myin','on','Ground','');
      |     InputConnector('Mzin','on','Ground','');
      | end
      mask TypeOptions VDeflectionTypePanel: Simple spring and damper | External
      mask Callback VDeflectionTypePanel:
      | maskObj = Simulink.Mask.get(gcb);
      | 
      | Type_tmp = maskObj.getParameter('VDeflectionTypePanel');
      | Type     = Type_tmp.Value;
      | 
      | Group = maskObj.getDialogControl('VDeflectionModelGroup');
      | 
      | switch Type
      |     case 'Simple spring and damper'
      |     set_param([gcb,'/Contact model'],'LabelModeActiveChoice', 'Simple spring and damper');
      |     Group.Visible = 'on';
      |     InputConnector('Fzin','off','Ground','');
      |     case 'External'
      |     set_param([gcb,'/Contact model'],'LabelModeActiveChoice', 'External');
      |     Group.Visible = 'off';
      |     InputConnector('Fzin','on','Ground','');
      | end
      mask DialogControl BlockOptionsPanel Prompt: Block Options
      mask DialogControl FrictionModelPanel Prompt: Friction model
      mask DialogControl LinearTireModelGroup Prompt: Linear tire model
      mask DialogControl LinLongPanel Prompt: Longitudinal
      mask DialogControl LinLateralPanel Prompt: Lateral
      mask DialogControl BrakeSubPanel Prompt: Brake
      mask DialogControl BrakeGeneralGroup Prompt: General
      mask DialogControl BrakeDrumGroup Prompt: Drum Brake
      mask DialogControl BrakeDiscGroup Prompt: Disc Brake
      mask DialogControl BrakeMappedGroup Prompt: Mapped Brake
      mask DialogControl PlotBrakeTorqueMapButton Prompt: Plot brake torque map
      mask DialogControl PlotBrakeTorqueMapButton Callback:
      | maskObj = Simulink.Mask.get(gcb);
      | tmp = maskObj.getParameter('brake_p_bpt');
      | brake_p_bpt = str2num(tmp.Value);
      | tmp = maskObj.getParameter('brake_n_bpt');
      | brake_n_bpt = str2num(tmp.Value);
      | tmp = maskObj.getParameter('f_brake_t');
      | f_brake_t = str2num(tmp.Value);
      | 
      | figure;
      | surf(brake_p_bpt, brake_n_bpt, f_brake_t');
      | xlabel('Applied brake pressure [bar]');
      | ylabel('Wheel speed [rpm]');
      | zlabel('Brake torque [N*m]');
      | title('Brake torque vs applied pressure and wheel speed');
      mask DialogControl VDeflectionSubPanel Prompt: Vertical Deflection
      mask DialogControl VerticalModelGroup Prompt: Vertical deflection model
      mask DialogControl MassParameterPanel Prompt: Mass parameters
      mask DialogControl DimensionParameterPanel Prompt: Dimension parameters
      mask DialogControl InitialConditionPanel Prompt: Initial condition
  HubJoint_B : PMIOPort  Side=Left
  HubJoint_F : PMIOPort  Port=2  Side=Left
  Info : Outport
  Fx : Outport  Port=2
  Fy : Outport  Port=3
  Fz : Outport  Port=4
  Mx : Outport  Port=5
  My : Outport  Port=6
  Mz : Outport  Port=7

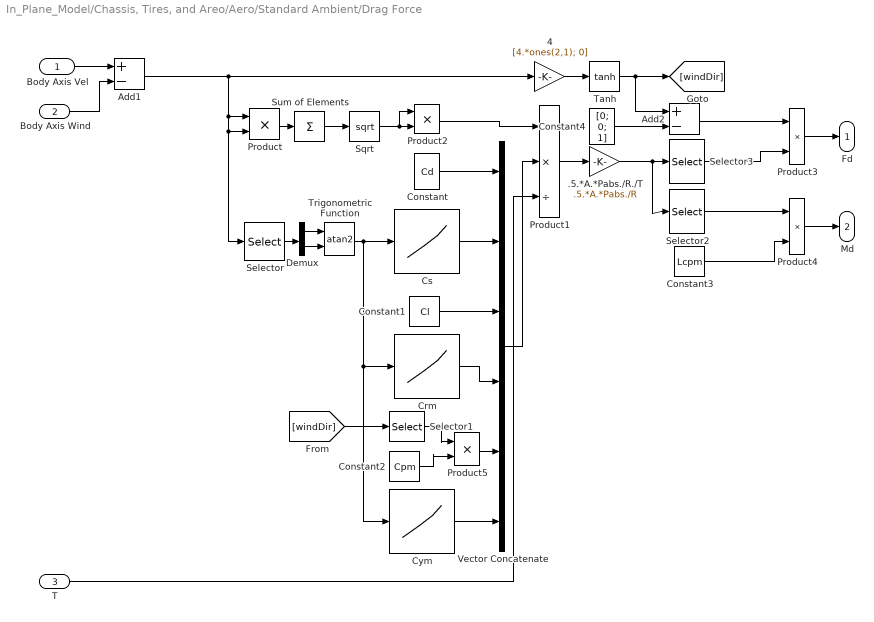
== system In_Plane_Model/Chassis, Tires, and Areo/Aero/Standard Ambient/Drag Force ==
  Body Axis Vel : Inport
  Body Axis Wind : Inport  Port=2
  T : Inport  Port=3  OutMin=1
  .5.*A.*Pabs./R./T : Gain  Gain=.5.*A.*Pabs./R
  4 : Gain  Gain=[4.*ones(2,1); 0]
  Add1 : Sum  Inputs=+-
  Add2 : Sum  Inputs=+-
  Constant : Constant  Value=Cd
  Constant1 : Constant  Value=Cl
  Constant2 : Constant  Value=Cpm
  Constant3 : Constant  Value=Lcpm
  Constant4 : Constant  Value=[0; 0; 1]
  Crm : Lookup_n-D  NumberOfTableDimensions=1  BreakpointsForDimension1=[-1 1]  Table=[0 0]  InternalRulePriority=Speed  RndMeth=Simplest
  Cs : Lookup_n-D  NumberOfTableDimensions=1  BreakpointsForDimension1=beta_w  Table=Cs  ExtrapMethod=Clip  InternalRulePriority=Speed  RndMeth=Simplest
  Cym : Lookup_n-D  NumberOfTableDimensions=1  BreakpointsForDimension1=beta_w  Table=Cym  InternalRulePriority=Speed  RndMeth=Simplest
  Demux : Demux  Outputs=2
  Product{,2..5} (5 alike) : Product
  Product1 : Product  Inputs=**/
  Selector : Selector  InputPortWidth=3  IndexOptions=Index vector (dialog)  Indices=[2 1]  OutputSizes=1
  Selector1 : Selector  InputPortWidth=3  IndexOptions=Index vector (dialog)  Indices=[1]  OutputSizes=1
  Selector2 : Selector  InputPortWidth=6  IndexOptions=Index vector (dialog)  Indices=[4:6]  OutputSizes=1
  Selector3 : Selector  InputPortWidth=6  IndexOptions=Index vector (dialog)  Indices=[1:3]  OutputSizes=1
  Sqrt : Sqrt
  Sum of Elements : Sum  Inputs=+
  Tanh : Trigonometry  Operator=tanh
  Trigonometric Function : Trigonometry  Operator=atan2  OutputSignalType=real
  Vector Concatenate : Concatenate  NumInputs=6
  Fd : Outport  VectorParamsAs1DForOutWhenUnconnected=off
  Md : Outport  Port=2  VectorParamsAs1DForOutWhenUnconnected=off
  wires:
  4/1 -> Tanh/1
  Trigonometric Function/1 -> Cs/1, Cym/1, Crm/1
  Demux/1 -> Trigonometric Function/1
  Demux/2 -> Trigonometric Function/2
  T/1 -> Product1/3
  Product2/1 -> Product1/1
  Vector Concatenate/1 -> Product1/2
  Product5/1 -> Vector Concatenate/5
  Selector1/1 -> Product5/1
  Constant2/1 -> Product5/2
  [windDir] -> Selector1/1
  Constant1/1 -> Vector Concatenate/3
  Selector3/1 -> Product3/2
  Constant3/1 -> Product4/2
  Selector2/1 -> Product4/1
  Product4/1 -> Md/1
  Crm/1 -> Vector Concatenate/4
  Cym/1 -> Vector Concatenate/6
  Cs/1 -> Vector Concatenate/2
  Selector/1 -> Demux/1
  Product3/1 -> Fd/1
  Product/1 -> Sum of Elements/1
  Sum of Elements/1 -> Sqrt/1
  Sqrt/1 -> Product2/2, Product2/1
  .5.*A.*Pabs./R./T/1 -> Selector2/1, Selector3/1
  Constant/1 -> Vector Concatenate/1
  Product1/1 -> .5.*A.*Pabs./R./T/1
  Body Axis Vel/1 -> Add1/1
  Body Axis Wind/1 -> Add1/2
  Tanh/1 -> Add2/1, [windDir]
  Add1/1 -> 4/1, Product/1, Product/2, Selector/1
  Add2/1 -> Product3/1
  Constant4/1 -> Add2/2

== system In_Plane_Model/Chassis, Tires, and Areo/Aero/Standard Ambient/Sensor_Frm ==
  PS-Simulink Converter1 : nesl_utility_internal/PS-Simulink Converter  PhysicalDomain=network_engine_domain  SubClassName=ps_output  LeftPortType=input  RightPortType=output  PseudoPeriodic=off  Frequencies=[]  VectorFormat=1-D array  Unit=inherit  AffineConversion=off
  PS-Simulink Converter4 : nesl_utility_internal/PS-Simulink Converter  PhysicalDomain=network_engine_domain  SubClassName=ps_output  LeftPortType=input  RightPortType=output  PseudoPeriodic=off  Frequencies=[]  VectorFormat=1-D array  Unit=inherit  AffineConversion=off
  PS-Simulink Converter5 : nesl_utility_internal/PS-Simulink Converter  PhysicalDomain=network_engine_domain  SubClassName=ps_output  LeftPortType=input  RightPortType=output  PseudoPeriodic=off  Frequencies=[]  VectorFormat=1-D array  Unit=inherit  AffineConversion=off
  Transform Sensor1 : sm_lib/Frames and Transforms/Transform Sensor  MeasurementFrame=NonRotatingFollower  RotationSequence=XYX  SenseAngle=off  SenseAxis=off  SenseQ=off  SenseR=off  SenseRotationSequence=off  SenseOmegaX=off  SenseOmegaY=off  SenseOmegaZ=off  SenseOmega=off  SenseQDot=off  SenseRDot=off  SenseRotationSequenceDot=off  SenseAlphaX=off  SenseAlphaY=off  SenseAlphaZ=off  SenseAlpha=off  SenseQDDot=off  SenseRDDot=off  SenseX=off  SenseY=off  SenseZ=off  SenseXYZ=off  SenseRad=off  SenseAzim=off  SenseDist=off  SenseInc=off  SenseXDot=on  SenseYDot=on  SenseZDot=on  SenseXYZDot=off  SenseRadDot=off  SenseAzimDot=off  SenseDistDot=off  SenseIncDot=off  SenseXDDot=off  SenseYDDot=off  SenseZDDot=off  SenseXYZDDot=off  SenseRadDDot=off  SenseAzimDDot=off  SenseDistDDot=off  SenseIncDDot=off
  World Frame : sm_lib/Frames and Transforms/World Frame
  F : PMIOPort  Side=Left
  Vx_vf : Outport
  Vy_vf : Outport  Port=2
  Vz_vf : Outport  Port=3
  wires:
  PS-Simulink Converter1/1 -> Vz_vf/1
  PS-Simulink Converter4/1 -> Vx_vf/1
  PS-Simulink Converter5/1 -> Vy_vf/1
  connections:
  PS-Simulink Converter1/LConn1 -- Transform Sensor1/RConn4
  PS-Simulink Converter4/LConn1 -- Transform Sensor1/RConn2
  PS-Simulink Converter5/LConn1 -- Transform Sensor1/RConn3
  Transform Sensor1/RConn1 -- F/RConn1
  World Frame/RConn1 -- Transform Sensor1/LConn1

== system In_Plane_Model/Chassis, Tires, and Areo/Aero/Standard Ambient/rotation ==
  X : Inport  Partition=on  PartitionDimension=2  PartitionWidth=1  PartitionOffset=0
  theta : Inport  Port=2  Partition=on  PartitionDimension=1  PartitionWidth=1  PartitionOffset=0
  For Each : ForEach  DisableCoverage=on
  Mux2 : Mux  Inputs=3
  Rotation Angles to Direction Cosine Matrix : sharedtransform/Rotation Angles to Direction Cosine Matrix  rotationOrder=ZYX  aMode=aMode
  Selector1 : Selector  InputPortWidth=3  IndexOptions=Index vector (dialog)  Indices=[3 2 1]  OutputSizes=1
  Transpose1 : Math  Operator=transpose  SignedPower=on
  phi : Constant  Value=0
  psi : Constant  Value=0
  transform to body axes : shared6dof/6DOF (Euler Angles)/transform to Inertial axes   SystemSampleTime=-1  VariantActivationTime=update diagram  EmptyChoice=off  PassThrough=off  PassThroughVariantControl=(default)  EmptyChoiceVariantControl=(default)  AllowFlexibleInterface=on  Latency=0  AutoFrameSizeCalculation=off
  x : Outport  ConcatenationDimension=2  VectorParamsAs1DForOutWhenUnconnected=off
  wires:
  Transpose1/1 -> transform to body axes/2
  Selector1/1 -> Rotation Angles to Direction Cosine Matrix/1
  Mux2/1 -> Selector1/1
  Rotation Angles to Direction Cosine Matrix/1 -> Transpose1/1
  psi/1 -> Mux2/3
  phi/1 -> Mux2/1
  theta/1 -> Mux2/2
  transform to body axes/1 -> x/1
  X/1 -> transform to body axes/1
